simulink model "debouncerSimple"  (Simulink 7.2)
settings: Solver=VariableStepDiscrete  StartTime=0.0  StopTime=10  RelTol=1e-3
settings Model: Creator=mehran  LastModifiedBy=jrivitus
settings OptimizationCC: InitFltsAndDblsToZero=on  EfficientMapNaN2IntZero=off
settings DebuggingCC: SaveWithParameterizedLinksMsg=none  SignalResolutionControl=TryResolveAllWithWarning  MultiTaskDSMMsg=warning  MultiTaskCondExecSysMsg=none  StrictBusMsg=None
settings RTWCC: IncludeERTFirstTime=on
settings GRTTargetCC: TargetFcnLib=ansi_tfl_tmw.mat

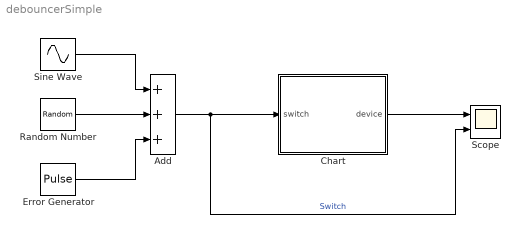
== system debouncerSimple ==
  Add : Sum  Inputs=+++  OutDataType=sfix(16)  OutScaling=2^-10
  Chart : Stateflow chart
  Error Generator : DiscretePulseGenerator  PulseType=Time based  Amplitude=10  Period=0.001  PulseWidth=50  PhaseDelay=2
  Random Number : RandomNumber  Variance=30  SampleTime=0
  Scope : Scope  NumInputPorts=2
      settings: TimeRange=10  YMin=-0.3~-40  YMax=1.3~50
  Sine Wave : Sin  Amplitude=20  Frequency=10  SampleTime=0
  wires:
  Sine Wave/1 -> Add/1
  Random Number/1 -> Add/2
  Error Generator/1 -> Add/3
  Chart/1(device) -> Scope/1
  Add/1 -> Scope/2, Chart/1(switch)  "Switch"

== stateflow chart Chart ==
  settings: updateMethod=DISCRETE  sampleTime=0.001
  state on
    entry: device = 1;
    state aboutToSwitch
      during: i++;
    state normal
      entry: i = 0;
    on.normal -> on.aboutToSwitch : [switch<0]
    on.aboutToSwitch -> on.normal : [switch>0]
    (default) -> on.normal
  state off
    entry: device = 0;
    state normal
      entry: i = 0;
    state aboutToSwitch
      during: i++;
    off.normal -> off.aboutToSwitch : [switch>0]
    (default) -> off.normal
    off.aboutToSwitch -> off.normal : [switch<0]
  (default) -> off
  off -> on : [i >= 40]
  on -> off : [i >= 40]
  data: k local int32 =0; device output boolean =0; i local int32 =0; switch input double
